simulink model "Unit_Step_Response"  (R2021b)
settings: Solver=VariableStepAuto  StartTime=0.0  StopTime=10.0  RelTol=1e-3
settings Model: Creator=Richi  LastModifiedBy=Richi

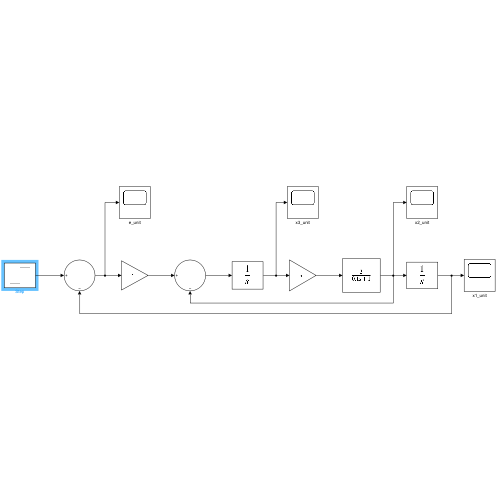
[thumbnail: Simulink's stored preview of the top-level diagram]
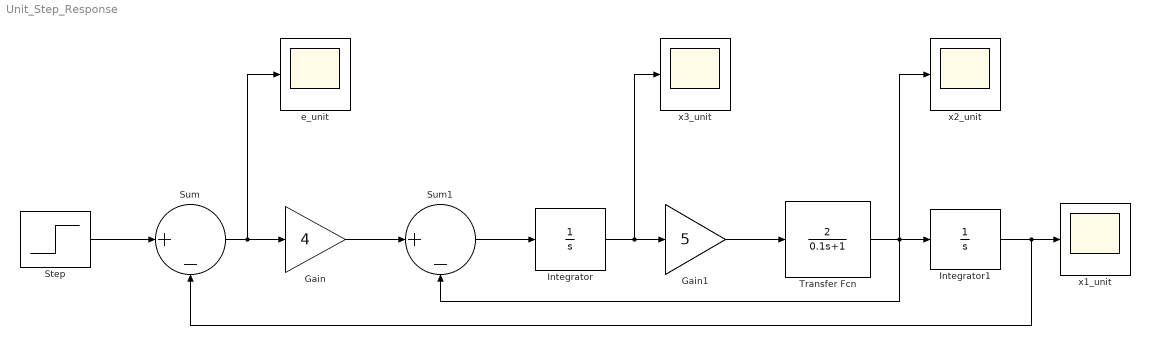
== system Unit_Step_Response ==
  Gain : Gain  Gain=4
  Gain1 : Gain  Gain=5
  Integrator : Integrator
  Integrator1 : Integrator
  Step : Step  SampleTime=0
  Sum : Sum  Inputs=|+-
  Sum1 : Sum  Inputs=|+-
  Transfer Fcn : TransferFcn  Numerator=[2]  Denominator=[0.1 1]
  e_unit : Scope
  x1_unit : Scope
  x2_unit : Scope
  x3_unit : Scope
  wires:
  Step/1 -> Sum/1
  Sum/1 -> Gain/1, e_unit/1
  Gain/1 -> Sum1/1
  Sum1/1 -> Integrator/1
  Integrator/1 -> x3_unit/1, Gain1/1
  Gain1/1 -> Transfer Fcn/1
  Transfer Fcn/1 -> Sum1/2, x2_unit/1, Integrator1/1
  Integrator1/1 -> Sum/2, x1_unit/1
